simulink model "double_pendulum_dynamics_controlled"  (R2020b)
settings: Solver=VariableStepAuto  StartTime=0.0  StopTime=7  RelTol=1e-3
libraries: simulink x2
settings Model: Creator=maximilianstoelzle  LastModifiedBy=maximilianstoelzle

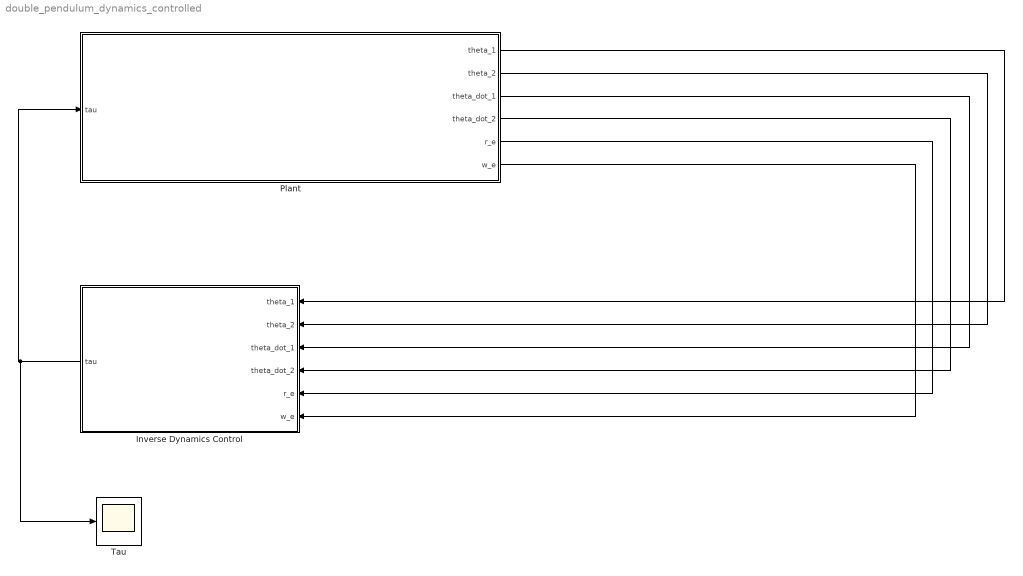
== system double_pendulum_dynamics_controlled ==
  Inverse Dynamics Control : MATLAB Function  TreatAsAtomicUnit=on
  Plant : Subsystem
  Tau : Scope
  wires:
  Inverse Dynamics Control/1(tau) -> Tau/1, Plant/1(tau)
  Plant/1(theta_1) -> Inverse Dynamics Control/1(theta_1)
  Plant/2(theta_2) -> Inverse Dynamics Control/2(theta_2)
  Plant/3(theta_dot_1) -> Inverse Dynamics Control/3(theta_dot_1)
  Plant/4(theta_dot_2) -> Inverse Dynamics Control/4(theta_dot_2)
  Plant/5(r_e) -> Inverse Dynamics Control/5(r_e)
  Plant/6(w_e) -> Inverse Dynamics Control/6(w_e)

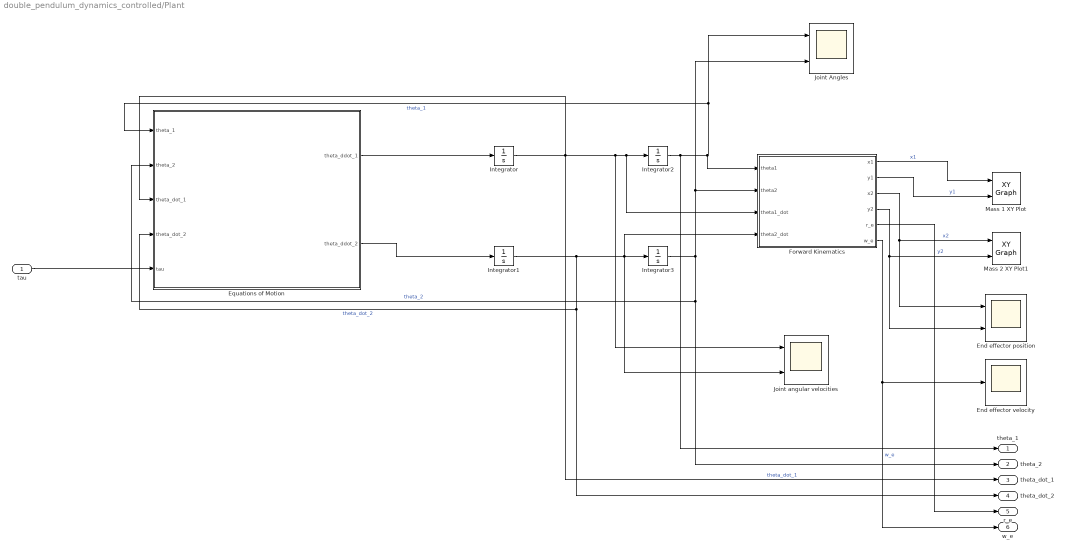
== system double_pendulum_dynamics_controlled/Plant ==
  tau : Inport
  End effector position : Scope  NumInputPorts=2
  End effector velocity : Scope
  Equations of Motion : MATLAB Function  TreatAsAtomicUnit=on
  Forward Kinematics : MATLAB Function  TreatAsAtomicUnit=on
  Integrator : Integrator
  Integrator1 : Integrator
  Integrator2 : Integrator
  Integrator3 : Integrator  InitialCondition=pi/2
  Joint Angles : Scope  NumInputPorts=2
  Joint angular velocities : Scope  NumInputPorts=2
  Mass 1 XY Plot : simulink/Sinks/XY Graph  xmin=-0.6  xmax=0.6  ymin=-0.6  ymax=0.6  st=-1
  Mass 2 XY Plot1 : simulink/Sinks/XY Graph  xmin=-1.6  xmax=1.6  ymin=-1.6  ymax=1.6  st=-1
  theta_1 : Outport
  theta_2 : Outport  Port=2
  theta_dot_1 : Outport  Port=3
  theta_dot_2 : Outport  Port=4
  r_e : Outport  Port=5
  w_e : Outport  Port=6
  wires:
  Forward Kinematics/4(y2) -> End effector position/2, Mass 2 XY Plot1/2  "y2"
  Forward Kinematics/5(r_e) -> r_e/1
  Integrator2/1 -> theta_1/1, Forward Kinematics/1(theta1), Equations of Motion/1(theta_1), Joint Angles/1  "theta_1"
  Forward Kinematics/1(x1) -> Mass 1 XY Plot/1  "x1"
  tau/1 -> Equations of Motion/5(tau)
  Equations of Motion/2(theta_ddot_2) -> Integrator1/1
  Integrator3/1 -> theta_2/1, Equations of Motion/2(theta_2), Forward Kinematics/2(theta2), Joint Angles/2  "theta_2"
  Integrator/1 -> theta_dot_1/1, Equations of Motion/3(theta_dot_1), Joint angular velocities/1, Forward Kinematics/3(theta1_dot), Integrator2/1  "theta_dot_1"
  Forward Kinematics/3(x2) -> End effector position/1, Mass 2 XY Plot1/1  "x2"
  Forward Kinematics/6(w_e) -> End effector velocity/1, w_e/1  "w_e"
  Forward Kinematics/2(y1) -> Mass 1 XY Plot/2  "y1"
  Equations of Motion/1(theta_ddot_1) -> Integrator/1
  Integrator1/1 -> Equations of Motion/4(theta_dot_2), theta_dot_2/1, Forward Kinematics/4(theta2_dot), Joint angular velocities/2, Integrator3/1  "theta_dot_2"

== matlab function double_pendulum_dynamics_controlled/Plant/Forward Kinematics ==
  data: theta1 input; x1 output; theta2 input; y1 output; x2 output; y2 output; r_e output; w_e output; theta1_dot input; theta2_dot input
function [x1, y1, x2, y2, r_e, w_e] = forward_kinematics(theta1, theta2, theta1_dot, theta2_dot)
    % parameters
    l1 = 0.5;
    l2 = 1;
    
    x1 = sin(theta1) * l1;
    y1 = -cos(theta1) * l1;
    
    x2 = x1 + sin(theta2) * l2;
    y2 = y1 - cos(theta2) * l2;
    r_e = [x2; y2];
    
    q_dot = [theta1_dot; theta2_dot];
    % geometric positional Jacobian
    J_eP = [cos(theta1) * l1, cos(theta2) * l2;
            sin(theta1) * l1, sin(theta2) * l2];
        
    w_e = J_eP * q_dot;

== matlab function double_pendulum_dynamics_controlled/Plant/Equations of Motion ==
  data: theta_1 input; theta_ddot_1 output; theta_2 input; theta_dot_1 input; theta_dot_2 input; theta_ddot_2 output; tau input
function [theta_ddot_1, theta_ddot_2]= EoM(theta_1, theta_2, theta_dot_1, theta_dot_2, tau)
    % parameters
    l = 1; % [m]
    acc_g = 9.81; % [m/s^2]
    lambda = 0.0001;
    
    M = [5/4, 1/2*cos(theta_1-theta_2); 1/2*cos(theta_1-theta_2), 1]*l;
    b = 1/2*l*sin(theta_1-theta_2)*[theta_dot_1^2; -theta_dot_2^2];
    g = acc_g*[sin(theta_1); sin(theta_2)];
    
    % q = [theta_1; theta_2];
    % q_dot = [theta_dot_1; theta_dot_2];
    q_ddot = pinv(M, lambda)*(tau - b - g);
    theta_ddot_1 = q_ddot(1);
    theta_ddot_2 = q_ddot(2);

== matlab function double_pendulum_dynamics_controlled/Inverse Dynamics Control ==
  data: theta_1 input; tau output; theta_2 input; theta_dot_1 input; theta_dot_2 input; r_e input; w_e input
function tau = inv_dynamics_control(theta_1, theta_2, theta_dot_1, theta_dot_2, r_e, w_e)
    r_e_des = [0; 1]; % desired end-effector position [m]
    w_e_des = [0; 0]; % desired end-effector task-space velocity [m/s]

    % parameters
    kp = 1; % proportional gain
    D = 0.8; % Damping ratio: D=1 => critical damping, D>1 => over critical damping
    kd = 2 * D * sqrt(kp); % damping gain
    l = 1; % [m]
    acc_g = 9.81; % [m/s^2]
    lambda = 0.0001;
    
    % desired end effector acceleration in task-space
    w_e_dot_des = kp * (r_e_des - r_e) + kd * (w_e_des - w_e);
    
    % joint angular velocity
    q_dot = [theta_dot_1; theta_dot_2];
    
    % geometric positional Jacobian
    J_eP = l*[1/2 * cos(theta_1), cos(theta_2); 1/2 * sin(theta_1), sin(theta_2)];
    % time-derivative of geometric positional Jacobian
    J_eP_dot = l*[-1/2*sin(theta_1)*theta_dot_1, -sin(theta_2)*theta_dot_2; 1/2*cos(theta_1)*theta_dot_1, cos(theta_2)*theta_dot_2];
    
    % compute desired generalized joint accelerations
    q_ddot_des = pinv(J_eP, lambda) * (w_e_dot_des - J_eP_dot * q_dot);
    
    % components of equation of motion
    M = [5/4, 1/2*cos(theta_1-theta_2); 1/2*cos(theta_1-theta_2), 1]*l;
    b = 1/2*l*sin(theta_1-theta_2)*[theta_dot_1^2; -theta_dot_2^2];
    g = acc_g*[sin(theta_1); sin(theta_2)];
    
    tau = M * q_ddot_des + b + g;
